simulink model "Adelanto_digital_tarea"  (R2020a)
settings: Solver=ode45  StartTime=0.0  StopTime=10  MaxStep=1e-5  RelTol=1e-3  EnableMultiTasking=on
values from neighbouring files (symbols this model uses):
  T = 0.2    [Ejemplo1.m]    (also in Tito_Ricardo_Tarea_2_Ad.m = 0.23; Tito_Ricardo_Tarea_2_At.m = 0.23; Tito_Ricardo_Tarea_2_PD.m = 0.23; Tito_Ricardo_Tarea_2_PI.m = 0.23)
settings Model: Creator=Usuario  LastModifiedBy=Usuario
settings DataIOCC: SaveFormat=Array  SignalLoggingSaveFormat=ModelDataLogs  ReturnWorkspaceOutputs=off
settings OptimizationCC: InitFltsAndDblsToZero=on  LifeSpan=inf
settings DebuggingCC: SaveWithParameterizedLinksMsg=none  UnderspecifiedInitializationDetection=Classic  MergeDetectMultiDrivingBlocksExec=none  SignalResolutionControl=TryResolveAllWithWarning  SolverPrmCheckMsg=warning  MultiTaskDSMMsg=warning  MultiTaskCondExecSysMsg=none  FcnCallInpInsideContextMsg=warning  SFUnexpectedBacktrackingDiag=warning  SFNoUnconditionalDefaultTransitionDiag=warning  SFExecutionAtInitializationDiag=none  ArithmeticOperatorsInVariantConditions=warning
settings HardwareCC: ProdBitPerPointer=32  ProdBitPerSizeT=32  ProdBitPerPtrDiffT=32  ProdLargestAtomicFloat=None  ProdIntDivRoundTo=Undefined  ProdEndianess=Unspecified  ProdWordSize=32  ProdHWDeviceType=32-bit Generic
settings ModelReferenceCC: PropagateSignalLabelsOutOfModel=off
settings SFSimCC: SimUseLocalCustomCode=off  CustomCodeUndefinedFunction=UseInterfaceOnly
settings RTWCC: RTWUseLocalCustomCode=off
settings CodeAppCC: StateflowObjectComments=on
settings GRTTargetCC: TargetFcnLib=ansi_tfl_tmw.mat  TargetLangStandard=C89/C90 (ANSI)  CombineOutputUpdateFcns=off  GRTInterface=on
settings ConfigComp: CovMetricSettings=dw  CovHtmlReporting=on  CovSaveCumulativeToWorkspaceVar=on  CovSaveSingleToWorkspaceVar=on  CovExternalEMLEnable=off  CovSFcnEnable=off

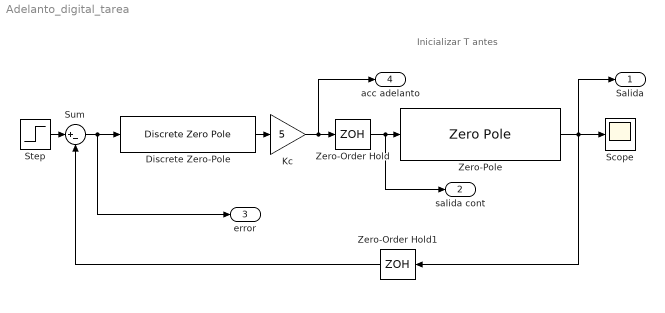
== system Adelanto_digital_tarea ==
  note: Inicializar T antes
  Discrete Zero-Pole : DiscreteZeroPole  Zeros=[0.003315]  Poles=[0.6313 0.6313]  Gain=1.705  SampleTime=-1
  Kc : Gain  Gain=5
  Scope : Scope
  Step : Step  Time=0  SampleTime=T
  Sum : Sum  Inputs=|+-
  Zero-Order Hold : ZeroOrderHold  SampleTime=T
  Zero-Order Hold1 : ZeroOrderHold  SampleTime=T
  Zero-Pole : ZeroPole  Zeros=[0.9794]  Poles=[0.003315]  Gain=0.14
  Salida : Outport
  salida cont : Outport  Port=2
  error : Outport  Port=3
  acc adelanto : Outport  Port=4
  wires:
  Zero-Order Hold/1 -> Zero-Pole/1, salida cont/1
  Step/1 -> Sum/1
  Zero-Pole/1 -> Salida/1, Zero-Order Hold1/1, Scope/1
  Zero-Order Hold1/1 -> Sum/2
  Sum/1 -> Discrete Zero-Pole/1, error/1
  Kc/1 -> Zero-Order Hold/1, acc adelanto/1
  Discrete Zero-Pole/1 -> Kc/1
